simulink model "BInverterError"  (R2024b)
settings: configuration reference "STM32H7_Config" (kept outside this file)
libraries: simulink x8
settings Model: DataDictionary=Master_Dictionary.sldd  EnableAccessToBaseWorkspace=off  Creator=torni  LastModifiedBy=Will
settings ConfigSetRef: SourceName=STM32H7_Config

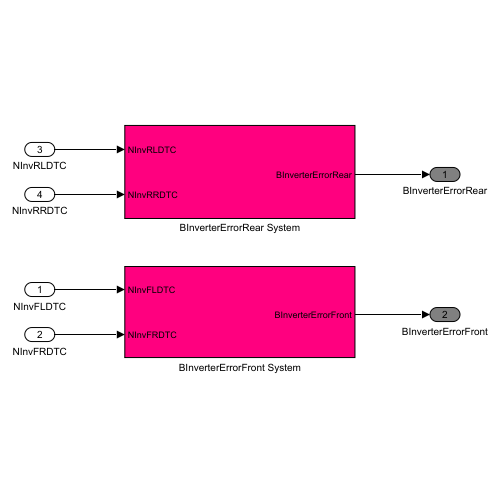
[thumbnail: Simulink's stored preview of the top-level diagram]
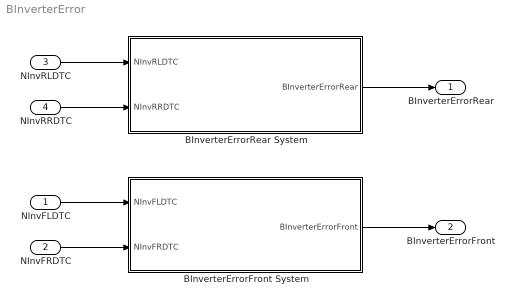
== system BInverterError ==
  NInvFLDTC : Inport  OutDataTypeStr=double
  NInvFRDTC : Inport  Port=2  OutDataTypeStr=double
  NInvRLDTC : Inport  Port=3  OutDataTypeStr=double
  NInvRRDTC : Inport  Port=4  OutDataTypeStr=double
  BInverterErrorFront System : Subsystem
  BInverterErrorRear System : Subsystem
  BInverterErrorRear : Outport  OutDataTypeStr=boolean  VectorParamsAs1DForOutWhenUnconnected=off
  BInverterErrorFront : Outport  Port=2  OutDataTypeStr=boolean  VectorParamsAs1DForOutWhenUnconnected=off
  wires:
  BInverterErrorFront System/1(BInverterErrorFront) -> BInverterErrorFront/1
  NInvRRDTC/1 -> BInverterErrorRear System/2(NInvRRDTC)
  NInvFLDTC/1 -> BInverterErrorFront System/1(NInvFLDTC)
  BInverterErrorRear System/1(BInverterErrorRear) -> BInverterErrorRear/1
  NInvFRDTC/1 -> BInverterErrorFront System/2(NInvFRDTC)
  NInvRLDTC/1 -> BInverterErrorRear System/1(NInvRLDTC)

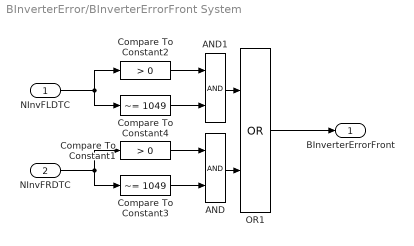
== system BInverterError/BInverterErrorFront System ==
  NInvFLDTC : Inport  OutDataTypeStr=double
  NInvFRDTC : Inport  Port=2  OutDataTypeStr=double
  AND : Logic  AllPortsSameDT=off  OutDataTypeStr=boolean
  AND1 : Logic  AllPortsSameDT=off  OutDataTypeStr=boolean
  Compare To Constant1 : simulink/Logic and Bit Operations/Compare To Constant  relop=>  const=0  OutDataTypeStr=boolean
  Compare To Constant2 : simulink/Logic and Bit Operations/Compare To Constant  relop=>  const=0  OutDataTypeStr=boolean
  Compare To Constant3 : simulink/Logic and Bit Operations/Compare To Constant  relop=~=  const=1049  OutDataTypeStr=boolean
  Compare To Constant4 : simulink/Logic and Bit Operations/Compare To Constant  relop=~=  const=1049  OutDataTypeStr=boolean
  OR1 : Logic  Operator=OR  AllPortsSameDT=off  OutDataTypeStr=boolean
  BInverterErrorFront : Outport  OutDataTypeStr=boolean  VectorParamsAs1DForOutWhenUnconnected=off
  wires:
  OR1/1 -> BInverterErrorFront/1
  Compare To Constant2/1 -> AND1/1
  Compare To Constant1/1 -> AND/1
  NInvFLDTC/1 -> Compare To Constant2/1, Compare To Constant4/1
  Compare To Constant3/1 -> AND/2
  Compare To Constant4/1 -> AND1/2
  NInvFRDTC/1 -> Compare To Constant3/1, Compare To Constant1/1
  AND1/1 -> OR1/1
  AND/1 -> OR1/2

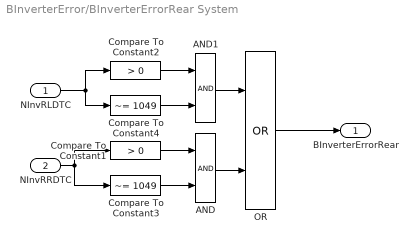
== system BInverterError/BInverterErrorRear System ==
  NInvRLDTC : Inport  OutDataTypeStr=double
  NInvRRDTC : Inport  Port=2  OutDataTypeStr=double
  AND : Logic  AllPortsSameDT=off  OutDataTypeStr=boolean
  AND1 : Logic  AllPortsSameDT=off  OutDataTypeStr=boolean
  Compare To Constant1 : simulink/Logic and Bit Operations/Compare To Constant  relop=>  const=0  OutDataTypeStr=boolean
  Compare To Constant2 : simulink/Logic and Bit Operations/Compare To Constant  relop=>  const=0  OutDataTypeStr=boolean
  Compare To Constant3 : simulink/Logic and Bit Operations/Compare To Constant  relop=~=  const=1049  OutDataTypeStr=boolean
  Compare To Constant4 : simulink/Logic and Bit Operations/Compare To Constant  relop=~=  const=1049  OutDataTypeStr=boolean
  OR : Logic  Operator=OR  AllPortsSameDT=off  OutDataTypeStr=boolean
  BInverterErrorRear : Outport  OutDataTypeStr=boolean  VectorParamsAs1DForOutWhenUnconnected=off
  wires:
  OR/1 -> BInverterErrorRear/1
  AND1/1 -> OR/1
  Compare To Constant3/1 -> AND/2
  AND/1 -> OR/2
  Compare To Constant1/1 -> AND/1
  NInvRRDTC/1 -> Compare To Constant3/1, Compare To Constant1/1
  Compare To Constant2/1 -> AND1/1
  Compare To Constant4/1 -> AND1/2
  NInvRLDTC/1 -> Compare To Constant4/1, Compare To Constant2/1
